simulink model "SIMULINKcommande_adaptative_parm_connus2018b"  (R2018b)
settings: Solver=VariableStepAuto  StartTime=0.0  StopTime=10  RelTol=1e-3
settings Model: Creator=PC  LastModifiedBy=PC
settings DataIOCC: ReturnWorkspaceOutputs=on

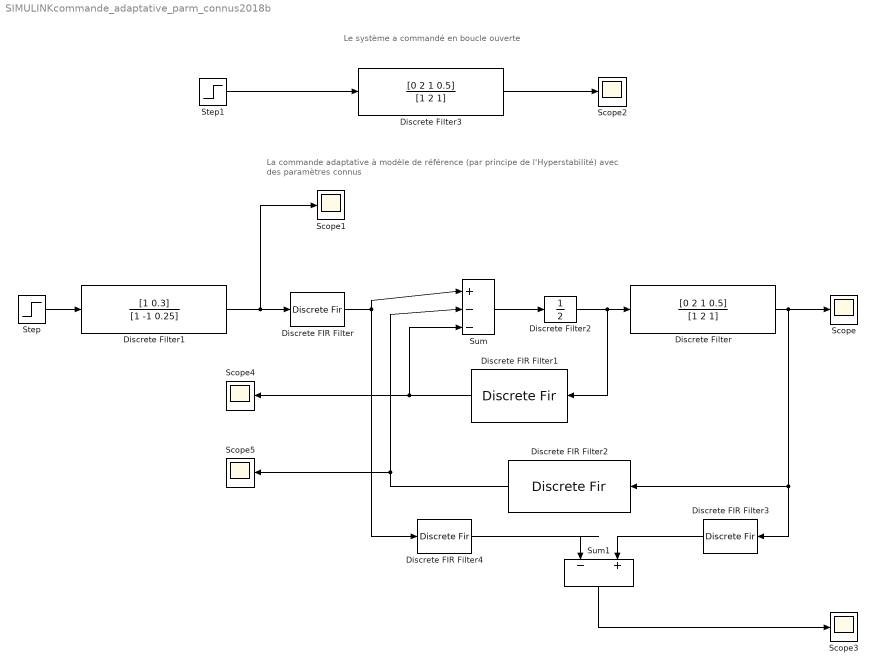
== system SIMULINKcommande_adaptative_parm_connus2018b ==
  note: La commande adaptative à modèle de référence (par principe de l'Hyperstabilité)
      | avec des paramètres connus
  note: Le système a commandé en boucle ouverte
  Discrete FIR Filter : DiscreteFir  Coefficients=[1 0.5]  SampleTime=0.1
  Discrete FIR Filter1 : DiscreteFir  Coefficients=[0 1 0.5]  SampleTime=0.1
  Discrete FIR Filter2 : DiscreteFir  Coefficients=[-1.5 -1]  SampleTime=0.1
  Discrete FIR Filter3 : DiscreteFir  Coefficients=[1 0.5]  SampleTime=0.1
  Discrete FIR Filter4 : DiscreteFir  Coefficients=[0 1]  SampleTime=0.1
  Discrete Filter : DiscreteFilter  Numerator=[0 2 1 0.5]  Denominator=[1 2 1]  InitialStates=1  InitialDenominatorStates=[1 1]  SampleTime=0.1
  Discrete Filter1 : DiscreteFilter  Numerator=[1 0.3]  Denominator=[1 -1 0.25]  InitialStates=2  SampleTime=0.1
  Discrete Filter2 : DiscreteFilter  Numerator=1  Denominator=2  SampleTime=.1
  Discrete Filter3 : DiscreteFilter  Numerator=[0 2 1 0.5]  Denominator=[1 2 1]  InitialStates=1  SampleTime=0.1
  Scope{,1..5} (6 alike) : Scope
  Step : Step  Time=0  SampleTime=0
  Step1 : Step  SampleTime=0
  Sum : Sum  Inputs=|+--
  Sum1 : Sum  Inputs=|-+
  wires:
  Discrete Filter1/1 -> Discrete FIR Filter/1, Scope1/1
  Discrete FIR Filter/1 -> Sum/1, Discrete FIR Filter4/1
  Discrete Filter2/1 -> Discrete FIR Filter1/1, Discrete Filter/1
  Sum/1 -> Discrete Filter2/1
  Step/1 -> Discrete Filter1/1
  Discrete Filter/1 -> Discrete FIR Filter3/1, Discrete FIR Filter2/1, Scope/1
  Discrete FIR Filter2/1 -> Scope5/1, Sum/2
  Discrete FIR Filter1/1 -> Scope4/1, Sum/3
  Step1/1 -> Discrete Filter3/1
  Discrete Filter3/1 -> Scope2/1
  Sum1/1 -> Scope3/1
  Discrete FIR Filter3/1 -> Sum1/2
  Discrete FIR Filter4/1 -> Sum1/1
